simulink model "RADTRANS003"  (R2020b)
settings: Solver=VariableStepAuto  StartTime=0.0  StopTime=10.0  RelTol=1e-3
undefined symbols (not defined in the file): L_street, Line_110_C, Line_110_L, Line_110_R, Line_220_C, Line_220_L, Line_220_R, Line_35_C, Line_35_L, Line_35_R, Line_6_L, Line_6_R, P_nom_dyn, Q_nom_dyn, R_street, Sys_f_Hz, Sys_V_net_kV, Tr_110_35_L_pu, Tr_110_35_R_pu, Tr_110_35_Sn_VA, Tr_110_35_V_HV_kV, Tr_110_35_V_LV_kV, Tr_110_6_L_pu, Tr_110_6_R_pu, Tr_110_6_Sn_VA, Tr_110_6_V_HV_kV, Tr_110_6_V_LV_kV, Tr_220_110_L_pu, Tr_220_110_R_pu, Tr_220_110_Sn_VA, Tr_220_110_V_HV_kV, Tr_220_110_V_LV_kV, Tr_35_04_L_pu, Tr_35_04_R_pu, Tr_35_04_Sn_VA, Tr_35_04_V_HV_kV, Tr_35_04_V_LV_kV, Tr_6_04_L_pu, Tr_6_04_R_pu, Tr_6_04_Sn_VA, Tr_6_04_V_HV_kV, Tr_6_04_V_LV_kV, Ts_powergui
libraries: dspstat3 x96, powerlib x81, powerlib_meascontrol x24, simulink x2
(part 2 of 3)

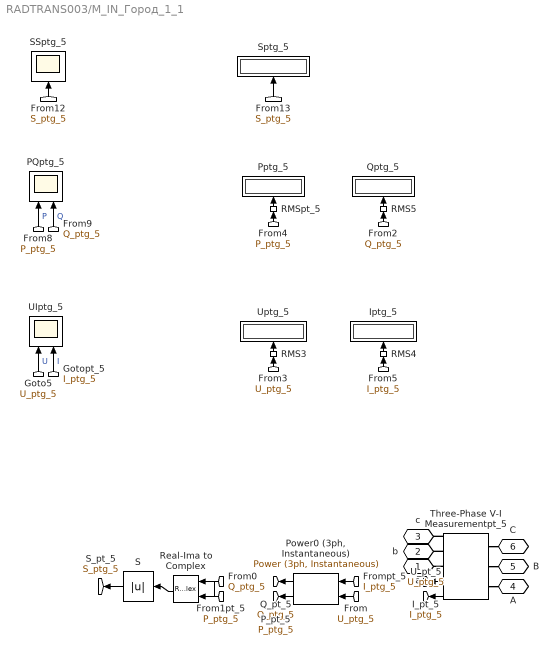
== system RADTRANS003/M_IN_Город_1_1 ==
  Iptg_5 : Display
      settings: Format=bank
  PQptg_5 : Scope  NumInputPorts=2
  "Power0 (3ph, Instantaneous)" : powerlib_meascontrol/Measurements/Power (3ph, Instantaneous)
  Pptg_5 : Display
      settings: Format=bank
  Qptg_5 : Display
      settings: Format=bank
  RMS3 : dspstat3/RMS  run=off  directionMode=Each column  dimension=1  InputProcessing=Columns as channels (frame based)  reset_popup=None
  RMS4 : dspstat3/RMS  run=off  directionMode=Each column  dimension=1  InputProcessing=Columns as channels (frame based)  reset_popup=None
  RMS5 : dspstat3/RMS  run=off  directionMode=Each column  dimension=1  InputProcessing=Columns as channels (frame based)  reset_popup=None
  RMSpt_5 : dspstat3/RMS  run=off  directionMode=Each column  dimension=1  InputProcessing=Columns as channels (frame based)  reset_popup=None
  Real-Ima to Complex : RealImagToComplex
  S : Abs
  SSptg_5 : Scope
  Sptg_5 : Display
      settings: Format=bank
  Three-Phase V-I Measurementpt_5 : powerlib/Measurements/Three-Phase V-I Measurement  VoltageMeasurement=phase-to-ground  SetLabelV=off  LabelV=Vabc  Vpu=off  VpuLL=off  CurrentMeasurement=yes  SetLabelI=off  LabelI=Iabc  Ipu=off  Pbase=100e6  Vbase=500e3  OutputType=Complex  PhasorSimulation=off  PSBequivalent=0
  UIptg_5 : Scope  NumInputPorts=2
  Uptg_5 : Display
      settings: Format=bank
  a : PMIOPort  Side=Right
  b : PMIOPort  Port=2  Side=Right
  c : PMIOPort  Port=3  Side=Right
  A : PMIOPort  Port=4  Side=Left
  B : PMIOPort  Port=5  Side=Left
  C : PMIOPort  Port=6  Side=Left
  tag scope: I_ptg_5=global, P_ptg_5=global, Q_ptg_5=global, S_ptg_5=global, U_ptg_5=global
  wires:
  S/1 -> [S_ptg_5]
  Real-Ima to Complex/1 -> S/1
  [S_ptg_5] -> Sptg_5/1
  [S_ptg_5] -> SSptg_5/1
  [P_ptg_5] -> RMSpt_5/1
  RMSpt_5/1 -> Pptg_5/1
  RMS5/1 -> Qptg_5/1
  [U_ptg_5] -> RMS3/1
  RMS3/1 -> Uptg_5/1
  [P_ptg_5] -> Real-Ima to Complex/1
  [Q_ptg_5] -> RMS5/1
  [I_ptg_5] -> RMS4/1
  RMS4/1 -> Iptg_5/1
  [U_ptg_5] -> UIptg_5/1  "U"
  [P_ptg_5] -> PQptg_5/1  "P"
  [I_ptg_5] -> UIptg_5/2  "I"
  Three-Phase V-I Measurementpt_5/1 -> [U_ptg_5]
  [Q_ptg_5] -> Real-Ima to Complex/2
  Three-Phase V-I Measurementpt_5/2 -> [I_ptg_5]
  [U_ptg_5] -> "Power0 (3ph, Instantaneous)"/1
  [I_ptg_5] -> "Power0 (3ph, Instantaneous)"/2
  "Power0 (3ph, Instantaneous)"/2 -> [Q_ptg_5]
  "Power0 (3ph, Instantaneous)"/1 -> [P_ptg_5]
  [Q_ptg_5] -> PQptg_5/2  "Q"
  connections:
  Three-Phase V-I Measurementpt_5/LConn1 -- A/RConn1
  Three-Phase V-I Measurementpt_5/RConn1 -- a/RConn1
  Three-Phase V-I Measurementpt_5/LConn2 -- B/RConn1
  Three-Phase V-I Measurementpt_5/LConn3 -- C/RConn1
  Three-Phase V-I Measurementpt_5/RConn3 -- c/RConn1
  Three-Phase V-I Measurementpt_5/RConn2 -- b/RConn1

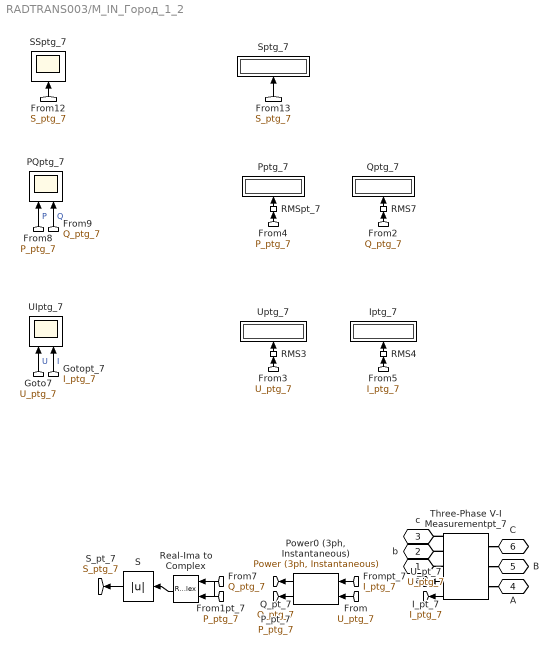
== system RADTRANS003/M_IN_Город_1_2 ==
  Iptg_7 : Display
      settings: Format=bank
  PQptg_7 : Scope  NumInputPorts=2
  "Power0 (3ph, Instantaneous)" : powerlib_meascontrol/Measurements/Power (3ph, Instantaneous)
  Pptg_7 : Display
      settings: Format=bank
  Qptg_7 : Display
      settings: Format=bank
  RMS3 : dspstat3/RMS  run=off  directionMode=Each column  dimension=1  InputProcessing=Columns as channels (frame based)  reset_popup=None
  RMS4 : dspstat3/RMS  run=off  directionMode=Each column  dimension=1  InputProcessing=Columns as channels (frame based)  reset_popup=None
  RMS7 : dspstat3/RMS  run=off  directionMode=Each column  dimension=1  InputProcessing=Columns as channels (frame based)  reset_popup=None
  RMSpt_7 : dspstat3/RMS  run=off  directionMode=Each column  dimension=1  InputProcessing=Columns as channels (frame based)  reset_popup=None
  Real-Ima to Complex : RealImagToComplex
  S : Abs
  SSptg_7 : Scope
  Sptg_7 : Display
      settings: Format=bank
  Three-Phase V-I Measurementpt_7 : powerlib/Measurements/Three-Phase V-I Measurement  VoltageMeasurement=phase-to-ground  SetLabelV=off  LabelV=Vabc  Vpu=off  VpuLL=off  CurrentMeasurement=yes  SetLabelI=off  LabelI=Iabc  Ipu=off  Pbase=100e6  Vbase=500e3  OutputType=Complex  PhasorSimulation=off  PSBequivalent=0
  UIptg_7 : Scope  NumInputPorts=2
  Uptg_7 : Display
      settings: Format=bank
  a : PMIOPort  Side=Right
  b : PMIOPort  Port=2  Side=Right
  c : PMIOPort  Port=3  Side=Right
  A : PMIOPort  Port=4  Side=Left
  B : PMIOPort  Port=5  Side=Left
  C : PMIOPort  Port=6  Side=Left
  tag scope: I_ptg_7=global, P_ptg_7=global, Q_ptg_7=global, S_ptg_7=global, U_ptg_7=global
  wires:
  S/1 -> [S_ptg_7]
  Real-Ima to Complex/1 -> S/1
  [S_ptg_7] -> Sptg_7/1
  [S_ptg_7] -> SSptg_7/1
  [P_ptg_7] -> RMSpt_7/1
  RMSpt_7/1 -> Pptg_7/1
  RMS7/1 -> Qptg_7/1
  [U_ptg_7] -> RMS3/1
  RMS3/1 -> Uptg_7/1
  [P_ptg_7] -> Real-Ima to Complex/1
  [Q_ptg_7] -> RMS7/1
  [I_ptg_7] -> RMS4/1
  RMS4/1 -> Iptg_7/1
  [U_ptg_7] -> UIptg_7/1  "U"
  [P_ptg_7] -> PQptg_7/1  "P"
  [I_ptg_7] -> UIptg_7/2  "I"
  Three-Phase V-I Measurementpt_7/1 -> [U_ptg_7]
  [Q_ptg_7] -> Real-Ima to Complex/2
  Three-Phase V-I Measurementpt_7/2 -> [I_ptg_7]
  [U_ptg_7] -> "Power0 (3ph, Instantaneous)"/1
  [I_ptg_7] -> "Power0 (3ph, Instantaneous)"/2
  "Power0 (3ph, Instantaneous)"/2 -> [Q_ptg_7]
  "Power0 (3ph, Instantaneous)"/1 -> [P_ptg_7]
  [Q_ptg_7] -> PQptg_7/2  "Q"
  connections:
  Three-Phase V-I Measurementpt_7/LConn1 -- A/RConn1
  Three-Phase V-I Measurementpt_7/RConn1 -- a/RConn1
  Three-Phase V-I Measurementpt_7/LConn2 -- B/RConn1
  Three-Phase V-I Measurementpt_7/LConn3 -- C/RConn1
  Three-Phase V-I Measurementpt_7/RConn3 -- c/RConn1
  Three-Phase V-I Measurementpt_7/RConn2 -- b/RConn1

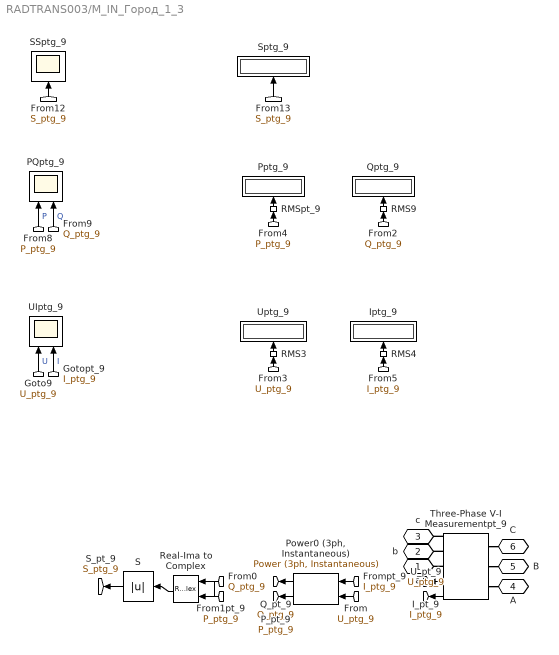
== system RADTRANS003/M_IN_Город_1_3 ==
  Iptg_9 : Display
      settings: Format=bank
  PQptg_9 : Scope  NumInputPorts=2
  "Power0 (3ph, Instantaneous)" : powerlib_meascontrol/Measurements/Power (3ph, Instantaneous)
  Pptg_9 : Display
      settings: Format=bank
  Qptg_9 : Display
      settings: Format=bank
  RMS3 : dspstat3/RMS  run=off  directionMode=Each column  dimension=1  InputProcessing=Columns as channels (frame based)  reset_popup=None
  RMS4 : dspstat3/RMS  run=off  directionMode=Each column  dimension=1  InputProcessing=Columns as channels (frame based)  reset_popup=None
  RMS9 : dspstat3/RMS  run=off  directionMode=Each column  dimension=1  InputProcessing=Columns as channels (frame based)  reset_popup=None
  RMSpt_9 : dspstat3/RMS  run=off  directionMode=Each column  dimension=1  InputProcessing=Columns as channels (frame based)  reset_popup=None
  Real-Ima to Complex : RealImagToComplex
  S : Abs
  SSptg_9 : Scope
  Sptg_9 : Display
      settings: Format=bank
  Three-Phase V-I Measurementpt_9 : powerlib/Measurements/Three-Phase V-I Measurement  VoltageMeasurement=phase-to-ground  SetLabelV=off  LabelV=Vabc  Vpu=off  VpuLL=off  CurrentMeasurement=yes  SetLabelI=off  LabelI=Iabc  Ipu=off  Pbase=100e6  Vbase=500e3  OutputType=Complex  PhasorSimulation=off  PSBequivalent=0
  UIptg_9 : Scope  NumInputPorts=2
  Uptg_9 : Display
      settings: Format=bank
  a : PMIOPort  Side=Right
  b : PMIOPort  Port=2  Side=Right
  c : PMIOPort  Port=3  Side=Right
  A : PMIOPort  Port=4  Side=Left
  B : PMIOPort  Port=5  Side=Left
  C : PMIOPort  Port=6  Side=Left
  tag scope: I_ptg_9=global, P_ptg_9=global, Q_ptg_9=global, S_ptg_9=global, U_ptg_9=global
  wires:
  S/1 -> [S_ptg_9]
  Real-Ima to Complex/1 -> S/1
  [S_ptg_9] -> Sptg_9/1
  [S_ptg_9] -> SSptg_9/1
  [P_ptg_9] -> RMSpt_9/1
  RMSpt_9/1 -> Pptg_9/1
  RMS9/1 -> Qptg_9/1
  [U_ptg_9] -> RMS3/1
  RMS3/1 -> Uptg_9/1
  [P_ptg_9] -> Real-Ima to Complex/1
  [Q_ptg_9] -> RMS9/1
  [I_ptg_9] -> RMS4/1
  RMS4/1 -> Iptg_9/1
  [U_ptg_9] -> UIptg_9/1  "U"
  [P_ptg_9] -> PQptg_9/1  "P"
  [I_ptg_9] -> UIptg_9/2  "I"
  Three-Phase V-I Measurementpt_9/1 -> [U_ptg_9]
  [Q_ptg_9] -> Real-Ima to Complex/2
  Three-Phase V-I Measurementpt_9/2 -> [I_ptg_9]
  [U_ptg_9] -> "Power0 (3ph, Instantaneous)"/1
  [I_ptg_9] -> "Power0 (3ph, Instantaneous)"/2
  "Power0 (3ph, Instantaneous)"/2 -> [Q_ptg_9]
  "Power0 (3ph, Instantaneous)"/1 -> [P_ptg_9]
  [Q_ptg_9] -> PQptg_9/2  "Q"
  connections:
  Three-Phase V-I Measurementpt_9/LConn1 -- A/RConn1
  Three-Phase V-I Measurementpt_9/RConn1 -- a/RConn1
  Three-Phase V-I Measurementpt_9/LConn2 -- B/RConn1
  Three-Phase V-I Measurementpt_9/LConn3 -- C/RConn1
  Three-Phase V-I Measurementpt_9/RConn3 -- c/RConn1
  Three-Phase V-I Measurementpt_9/RConn2 -- b/RConn1

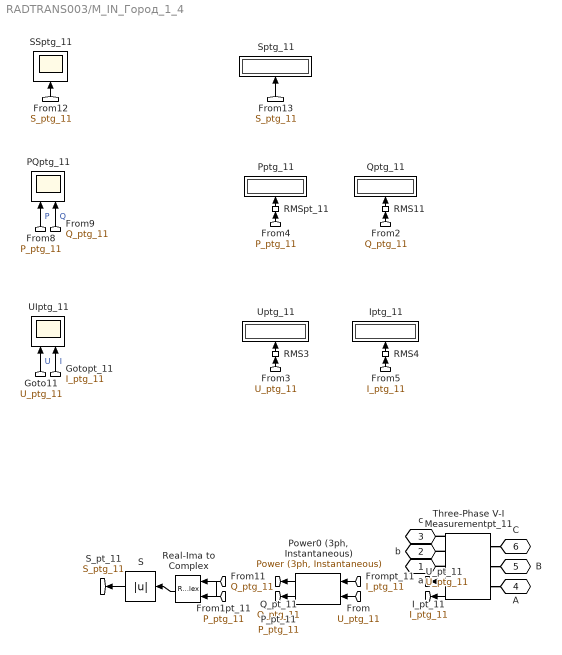
== system RADTRANS003/M_IN_Город_1_4 ==
  Iptg_11 : Display
      settings: Format=bank
  PQptg_11 : Scope  NumInputPorts=2
  "Power0 (3ph, Instantaneous)" : powerlib_meascontrol/Measurements/Power (3ph, Instantaneous)
  Pptg_11 : Display
      settings: Format=bank
  Qptg_11 : Display
      settings: Format=bank
  RMS11 : dspstat3/RMS  run=off  directionMode=Each column  dimension=1  InputProcessing=Columns as channels (frame based)  reset_popup=None
  RMS3 : dspstat3/RMS  run=off  directionMode=Each column  dimension=1  InputProcessing=Columns as channels (frame based)  reset_popup=None
  RMS4 : dspstat3/RMS  run=off  directionMode=Each column  dimension=1  InputProcessing=Columns as channels (frame based)  reset_popup=None
  RMSpt_11 : dspstat3/RMS  run=off  directionMode=Each column  dimension=1  InputProcessing=Columns as channels (frame based)  reset_popup=None
  Real-Ima to Complex : RealImagToComplex
  S : Abs
  SSptg_11 : Scope
  Sptg_11 : Display
      settings: Format=bank
  Three-Phase V-I Measurementpt_11 : powerlib/Measurements/Three-Phase V-I Measurement  VoltageMeasurement=phase-to-ground  SetLabelV=off  LabelV=Vabc  Vpu=off  VpuLL=off  CurrentMeasurement=yes  SetLabelI=off  LabelI=Iabc  Ipu=off  Pbase=100e6  Vbase=500e3  OutputType=Complex  PhasorSimulation=off  PSBequivalent=0
  UIptg_11 : Scope  NumInputPorts=2
  Uptg_11 : Display
      settings: Format=bank
  a : PMIOPort  Side=Right
  b : PMIOPort  Port=2  Side=Right
  c : PMIOPort  Port=3  Side=Right
  A : PMIOPort  Port=4  Side=Left
  B : PMIOPort  Port=5  Side=Left
  C : PMIOPort  Port=6  Side=Left
  tag scope: I_ptg_11=global, P_ptg_11=global, Q_ptg_11=global, S_ptg_11=global, U_ptg_11=global
  wires:
  S/1 -> [S_ptg_11]
  Real-Ima to Complex/1 -> S/1
  [S_ptg_11] -> Sptg_11/1
  [S_ptg_11] -> SSptg_11/1
  [P_ptg_11] -> RMSpt_11/1
  RMSpt_11/1 -> Pptg_11/1
  RMS11/1 -> Qptg_11/1
  [U_ptg_11] -> RMS3/1
  RMS3/1 -> Uptg_11/1
  [P_ptg_11] -> Real-Ima to Complex/1
  [Q_ptg_11] -> RMS11/1
  [I_ptg_11] -> RMS4/1
  RMS4/1 -> Iptg_11/1
  [U_ptg_11] -> UIptg_11/1  "U"
  [P_ptg_11] -> PQptg_11/1  "P"
  [I_ptg_11] -> UIptg_11/2  "I"
  Three-Phase V-I Measurementpt_11/1 -> [U_ptg_11]
  [Q_ptg_11] -> Real-Ima to Complex/2
  Three-Phase V-I Measurementpt_11/2 -> [I_ptg_11]
  [U_ptg_11] -> "Power0 (3ph, Instantaneous)"/1
  [I_ptg_11] -> "Power0 (3ph, Instantaneous)"/2
  "Power0 (3ph, Instantaneous)"/2 -> [Q_ptg_11]
  "Power0 (3ph, Instantaneous)"/1 -> [P_ptg_11]
  [Q_ptg_11] -> PQptg_11/2  "Q"
  connections:
  Three-Phase V-I Measurementpt_11/LConn1 -- A/RConn1
  Three-Phase V-I Measurementpt_11/RConn1 -- a/RConn1
  Three-Phase V-I Measurementpt_11/LConn2 -- B/RConn1
  Three-Phase V-I Measurementpt_11/LConn3 -- C/RConn1
  Three-Phase V-I Measurementpt_11/RConn3 -- c/RConn1
  Three-Phase V-I Measurementpt_11/RConn2 -- b/RConn1

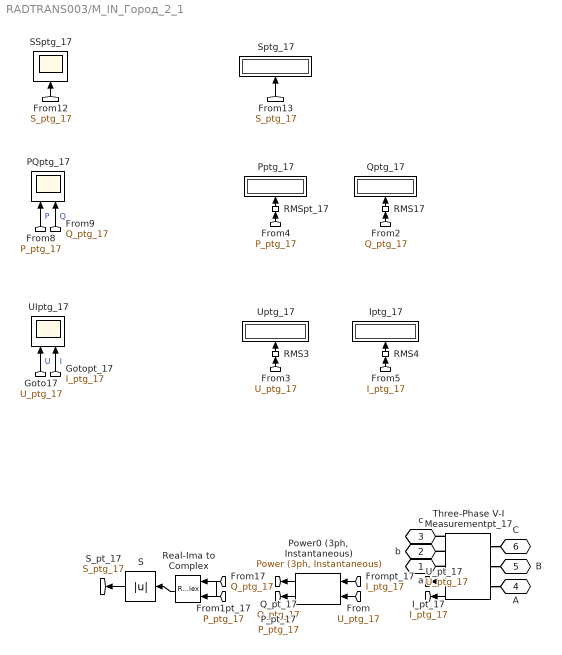
== system RADTRANS003/M_IN_Город_2_1 ==
  Iptg_17 : Display
      settings: Format=bank
  PQptg_17 : Scope  NumInputPorts=2
  "Power0 (3ph, Instantaneous)" : powerlib_meascontrol/Measurements/Power (3ph, Instantaneous)
  Pptg_17 : Display
      settings: Format=bank
  Qptg_17 : Display
      settings: Format=bank
  RMS17 : dspstat3/RMS  run=off  directionMode=Each column  dimension=1  InputProcessing=Columns as channels (frame based)  reset_popup=None
  RMS3 : dspstat3/RMS  run=off  directionMode=Each column  dimension=1  InputProcessing=Columns as channels (frame based)  reset_popup=None
  RMS4 : dspstat3/RMS  run=off  directionMode=Each column  dimension=1  InputProcessing=Columns as channels (frame based)  reset_popup=None
  RMSpt_17 : dspstat3/RMS  run=off  directionMode=Each column  dimension=1  InputProcessing=Columns as channels (frame based)  reset_popup=None
  Real-Ima to Complex : RealImagToComplex
  S : Abs
  SSptg_17 : Scope
  Sptg_17 : Display
      settings: Format=bank
  Three-Phase V-I Measurementpt_17 : powerlib/Measurements/Three-Phase V-I Measurement  VoltageMeasurement=phase-to-ground  SetLabelV=off  LabelV=Vabc  Vpu=off  VpuLL=off  CurrentMeasurement=yes  SetLabelI=off  LabelI=Iabc  Ipu=off  Pbase=100e6  Vbase=500e3  OutputType=Complex  PhasorSimulation=off  PSBequivalent=0
  UIptg_17 : Scope  NumInputPorts=2
  Uptg_17 : Display
      settings: Format=bank
  a : PMIOPort  Side=Right
  b : PMIOPort  Port=2  Side=Right
  c : PMIOPort  Port=3  Side=Right
  A : PMIOPort  Port=4  Side=Left
  B : PMIOPort  Port=5  Side=Left
  C : PMIOPort  Port=6  Side=Left
  tag scope: I_ptg_17=global, P_ptg_17=global, Q_ptg_17=global, S_ptg_17=global, U_ptg_17=global
  wires:
  S/1 -> [S_ptg_17]
  Real-Ima to Complex/1 -> S/1
  [S_ptg_17] -> Sptg_17/1
  [S_ptg_17] -> SSptg_17/1
  [P_ptg_17] -> RMSpt_17/1
  RMSpt_17/1 -> Pptg_17/1
  RMS17/1 -> Qptg_17/1
  [U_ptg_17] -> RMS3/1
  RMS3/1 -> Uptg_17/1
  [P_ptg_17] -> Real-Ima to Complex/1
  [Q_ptg_17] -> RMS17/1
  [I_ptg_17] -> RMS4/1
  RMS4/1 -> Iptg_17/1
  [U_ptg_17] -> UIptg_17/1  "U"
  [P_ptg_17] -> PQptg_17/1  "P"
  [I_ptg_17] -> UIptg_17/2  "I"
  Three-Phase V-I Measurementpt_17/1 -> [U_ptg_17]
  [Q_ptg_17] -> Real-Ima to Complex/2
  Three-Phase V-I Measurementpt_17/2 -> [I_ptg_17]
  [U_ptg_17] -> "Power0 (3ph, Instantaneous)"/1
  [I_ptg_17] -> "Power0 (3ph, Instantaneous)"/2
  "Power0 (3ph, Instantaneous)"/2 -> [Q_ptg_17]
  "Power0 (3ph, Instantaneous)"/1 -> [P_ptg_17]
  [Q_ptg_17] -> PQptg_17/2  "Q"
  connections:
  Three-Phase V-I Measurementpt_17/LConn1 -- A/RConn1
  Three-Phase V-I Measurementpt_17/RConn1 -- a/RConn1
  Three-Phase V-I Measurementpt_17/LConn2 -- B/RConn1
  Three-Phase V-I Measurementpt_17/LConn3 -- C/RConn1
  Three-Phase V-I Measurementpt_17/RConn3 -- c/RConn1
  Three-Phase V-I Measurementpt_17/RConn2 -- b/RConn1

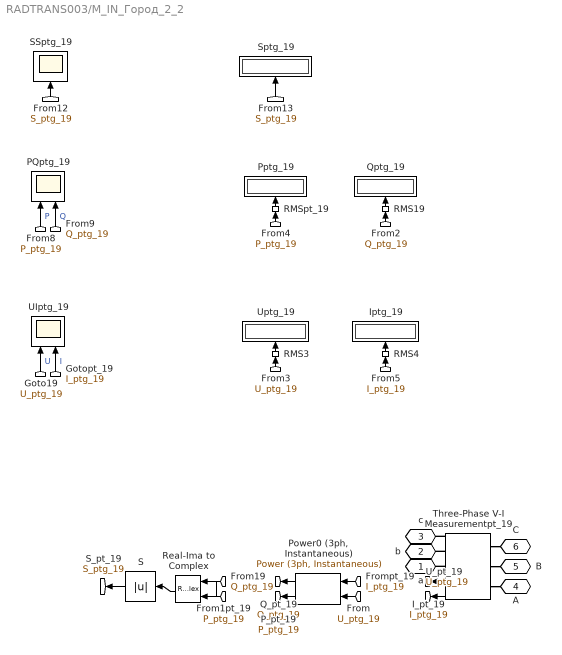
== system RADTRANS003/M_IN_Город_2_2 ==
  Iptg_19 : Display
      settings: Format=bank
  PQptg_19 : Scope  NumInputPorts=2
  "Power0 (3ph, Instantaneous)" : powerlib_meascontrol/Measurements/Power (3ph, Instantaneous)
  Pptg_19 : Display
      settings: Format=bank
  Qptg_19 : Display
      settings: Format=bank
  RMS19 : dspstat3/RMS  run=off  directionMode=Each column  dimension=1  InputProcessing=Columns as channels (frame based)  reset_popup=None
  RMS3 : dspstat3/RMS  run=off  directionMode=Each column  dimension=1  InputProcessing=Columns as channels (frame based)  reset_popup=None
  RMS4 : dspstat3/RMS  run=off  directionMode=Each column  dimension=1  InputProcessing=Columns as channels (frame based)  reset_popup=None
  RMSpt_19 : dspstat3/RMS  run=off  directionMode=Each column  dimension=1  InputProcessing=Columns as channels (frame based)  reset_popup=None
  Real-Ima to Complex : RealImagToComplex
  S : Abs
  SSptg_19 : Scope
  Sptg_19 : Display
      settings: Format=bank
  Three-Phase V-I Measurementpt_19 : powerlib/Measurements/Three-Phase V-I Measurement  VoltageMeasurement=phase-to-ground  SetLabelV=off  LabelV=Vabc  Vpu=off  VpuLL=off  CurrentMeasurement=yes  SetLabelI=off  LabelI=Iabc  Ipu=off  Pbase=100e6  Vbase=500e3  OutputType=Complex  PhasorSimulation=off  PSBequivalent=0
  UIptg_19 : Scope  NumInputPorts=2
  Uptg_19 : Display
      settings: Format=bank
  a : PMIOPort  Side=Right
  b : PMIOPort  Port=2  Side=Right
  c : PMIOPort  Port=3  Side=Right
  A : PMIOPort  Port=4  Side=Left
  B : PMIOPort  Port=5  Side=Left
  C : PMIOPort  Port=6  Side=Left
  tag scope: I_ptg_19=global, P_ptg_19=global, Q_ptg_19=global, S_ptg_19=global, U_ptg_19=global
  wires:
  S/1 -> [S_ptg_19]
  Real-Ima to Complex/1 -> S/1
  [S_ptg_19] -> Sptg_19/1
  [S_ptg_19] -> SSptg_19/1
  [P_ptg_19] -> RMSpt_19/1
  RMSpt_19/1 -> Pptg_19/1
  RMS19/1 -> Qptg_19/1
  [U_ptg_19] -> RMS3/1
  RMS3/1 -> Uptg_19/1
  [P_ptg_19] -> Real-Ima to Complex/1
  [Q_ptg_19] -> RMS19/1
  [I_ptg_19] -> RMS4/1
  RMS4/1 -> Iptg_19/1
  [U_ptg_19] -> UIptg_19/1  "U"
  [P_ptg_19] -> PQptg_19/1  "P"
  [I_ptg_19] -> UIptg_19/2  "I"
  Three-Phase V-I Measurementpt_19/1 -> [U_ptg_19]
  [Q_ptg_19] -> Real-Ima to Complex/2
  Three-Phase V-I Measurementpt_19/2 -> [I_ptg_19]
  [U_ptg_19] -> "Power0 (3ph, Instantaneous)"/1
  [I_ptg_19] -> "Power0 (3ph, Instantaneous)"/2
  "Power0 (3ph, Instantaneous)"/2 -> [Q_ptg_19]
  "Power0 (3ph, Instantaneous)"/1 -> [P_ptg_19]
  [Q_ptg_19] -> PQptg_19/2  "Q"
  connections:
  Three-Phase V-I Measurementpt_19/LConn1 -- A/RConn1
  Three-Phase V-I Measurementpt_19/RConn1 -- a/RConn1
  Three-Phase V-I Measurementpt_19/LConn2 -- B/RConn1
  Three-Phase V-I Measurementpt_19/LConn3 -- C/RConn1
  Three-Phase V-I Measurementpt_19/RConn3 -- c/RConn1
  Three-Phase V-I Measurementpt_19/RConn2 -- b/RConn1

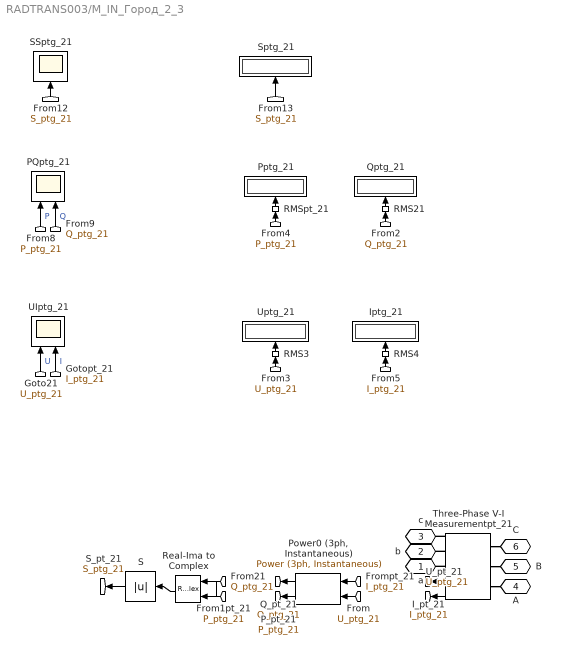
== system RADTRANS003/M_IN_Город_2_3 ==
  Iptg_21 : Display
      settings: Format=bank
  PQptg_21 : Scope  NumInputPorts=2
  "Power0 (3ph, Instantaneous)" : powerlib_meascontrol/Measurements/Power (3ph, Instantaneous)
  Pptg_21 : Display
      settings: Format=bank
  Qptg_21 : Display
      settings: Format=bank
  RMS21 : dspstat3/RMS  run=off  directionMode=Each column  dimension=1  InputProcessing=Columns as channels (frame based)  reset_popup=None
  RMS3 : dspstat3/RMS  run=off  directionMode=Each column  dimension=1  InputProcessing=Columns as channels (frame based)  reset_popup=None
  RMS4 : dspstat3/RMS  run=off  directionMode=Each column  dimension=1  InputProcessing=Columns as channels (frame based)  reset_popup=None
  RMSpt_21 : dspstat3/RMS  run=off  directionMode=Each column  dimension=1  InputProcessing=Columns as channels (frame based)  reset_popup=None
  Real-Ima to Complex : RealImagToComplex
  S : Abs
  SSptg_21 : Scope
  Sptg_21 : Display
      settings: Format=bank
  Three-Phase V-I Measurementpt_21 : powerlib/Measurements/Three-Phase V-I Measurement  VoltageMeasurement=phase-to-ground  SetLabelV=off  LabelV=Vabc  Vpu=off  VpuLL=off  CurrentMeasurement=yes  SetLabelI=off  LabelI=Iabc  Ipu=off  Pbase=100e6  Vbase=500e3  OutputType=Complex  PhasorSimulation=off  PSBequivalent=0
  UIptg_21 : Scope  NumInputPorts=2
  Uptg_21 : Display
      settings: Format=bank
  a : PMIOPort  Side=Right
  b : PMIOPort  Port=2  Side=Right
  c : PMIOPort  Port=3  Side=Right
  A : PMIOPort  Port=4  Side=Left
  B : PMIOPort  Port=5  Side=Left
  C : PMIOPort  Port=6  Side=Left
  tag scope: I_ptg_21=global, P_ptg_21=global, Q_ptg_21=global, S_ptg_21=global, U_ptg_21=global
  wires:
  S/1 -> [S_ptg_21]
  Real-Ima to Complex/1 -> S/1
  [S_ptg_21] -> Sptg_21/1
  [S_ptg_21] -> SSptg_21/1
  [P_ptg_21] -> RMSpt_21/1
  RMSpt_21/1 -> Pptg_21/1
  RMS21/1 -> Qptg_21/1
  [U_ptg_21] -> RMS3/1
  RMS3/1 -> Uptg_21/1
  [P_ptg_21] -> Real-Ima to Complex/1
  [Q_ptg_21] -> RMS21/1
  [I_ptg_21] -> RMS4/1
  RMS4/1 -> Iptg_21/1
  [U_ptg_21] -> UIptg_21/1  "U"
  [P_ptg_21] -> PQptg_21/1  "P"
  [I_ptg_21] -> UIptg_21/2  "I"
  Three-Phase V-I Measurementpt_21/1 -> [U_ptg_21]
  [Q_ptg_21] -> Real-Ima to Complex/2
  Three-Phase V-I Measurementpt_21/2 -> [I_ptg_21]
  [U_ptg_21] -> "Power0 (3ph, Instantaneous)"/1
  [I_ptg_21] -> "Power0 (3ph, Instantaneous)"/2
  "Power0 (3ph, Instantaneous)"/2 -> [Q_ptg_21]
  "Power0 (3ph, Instantaneous)"/1 -> [P_ptg_21]
  [Q_ptg_21] -> PQptg_21/2  "Q"
  connections:
  Three-Phase V-I Measurementpt_21/LConn1 -- A/RConn1
  Three-Phase V-I Measurementpt_21/RConn1 -- a/RConn1
  Three-Phase V-I Measurementpt_21/LConn2 -- B/RConn1
  Three-Phase V-I Measurementpt_21/LConn3 -- C/RConn1
  Three-Phase V-I Measurementpt_21/RConn3 -- c/RConn1
  Three-Phase V-I Measurementpt_21/RConn2 -- b/RConn1

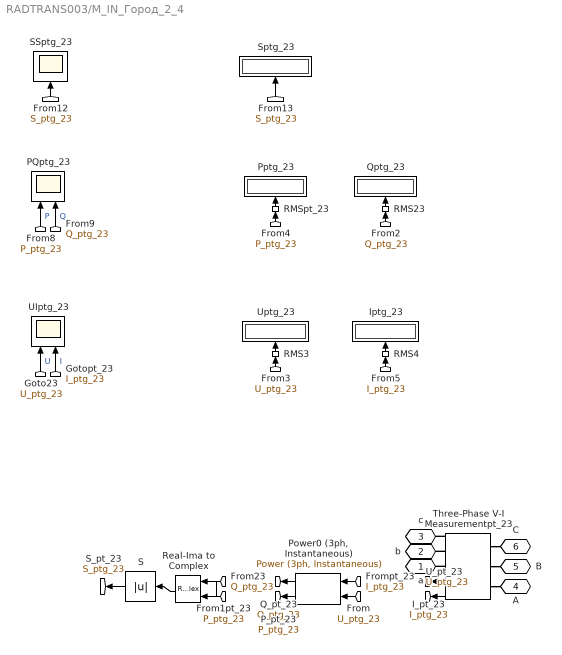
== system RADTRANS003/M_IN_Город_2_4 ==
  Iptg_23 : Display
      settings: Format=bank
  PQptg_23 : Scope  NumInputPorts=2
  "Power0 (3ph, Instantaneous)" : powerlib_meascontrol/Measurements/Power (3ph, Instantaneous)
  Pptg_23 : Display
      settings: Format=bank
  Qptg_23 : Display
      settings: Format=bank
  RMS23 : dspstat3/RMS  run=off  directionMode=Each column  dimension=1  InputProcessing=Columns as channels (frame based)  reset_popup=None
  RMS3 : dspstat3/RMS  run=off  directionMode=Each column  dimension=1  InputProcessing=Columns as channels (frame based)  reset_popup=None
  RMS4 : dspstat3/RMS  run=off  directionMode=Each column  dimension=1  InputProcessing=Columns as channels (frame based)  reset_popup=None
  RMSpt_23 : dspstat3/RMS  run=off  directionMode=Each column  dimension=1  InputProcessing=Columns as channels (frame based)  reset_popup=None
  Real-Ima to Complex : RealImagToComplex
  S : Abs
  SSptg_23 : Scope
  Sptg_23 : Display
      settings: Format=bank
  Three-Phase V-I Measurementpt_23 : powerlib/Measurements/Three-Phase V-I Measurement  VoltageMeasurement=phase-to-ground  SetLabelV=off  LabelV=Vabc  Vpu=off  VpuLL=off  CurrentMeasurement=yes  SetLabelI=off  LabelI=Iabc  Ipu=off  Pbase=100e6  Vbase=500e3  OutputType=Complex  PhasorSimulation=off  PSBequivalent=0
  UIptg_23 : Scope  NumInputPorts=2
  Uptg_23 : Display
      settings: Format=bank
  a : PMIOPort  Side=Right
  b : PMIOPort  Port=2  Side=Right
  c : PMIOPort  Port=3  Side=Right
  A : PMIOPort  Port=4  Side=Left
  B : PMIOPort  Port=5  Side=Left
  C : PMIOPort  Port=6  Side=Left
  tag scope: I_ptg_23=global, P_ptg_23=global, Q_ptg_23=global, S_ptg_23=global, U_ptg_23=global
  wires:
  S/1 -> [S_ptg_23]
  Real-Ima to Complex/1 -> S/1
  [S_ptg_23] -> Sptg_23/1
  [S_ptg_23] -> SSptg_23/1
  [P_ptg_23] -> RMSpt_23/1
  RMSpt_23/1 -> Pptg_23/1
  RMS23/1 -> Qptg_23/1
  [U_ptg_23] -> RMS3/1
  RMS3/1 -> Uptg_23/1
  [P_ptg_23] -> Real-Ima to Complex/1
  [Q_ptg_23] -> RMS23/1
  [I_ptg_23] -> RMS4/1
  RMS4/1 -> Iptg_23/1
  [U_ptg_23] -> UIptg_23/1  "U"
  [P_ptg_23] -> PQptg_23/1  "P"
  [I_ptg_23] -> UIptg_23/2  "I"
  Three-Phase V-I Measurementpt_23/1 -> [U_ptg_23]
  [Q_ptg_23] -> Real-Ima to Complex/2
  Three-Phase V-I Measurementpt_23/2 -> [I_ptg_23]
  [U_ptg_23] -> "Power0 (3ph, Instantaneous)"/1
  [I_ptg_23] -> "Power0 (3ph, Instantaneous)"/2
  "Power0 (3ph, Instantaneous)"/2 -> [Q_ptg_23]
  "Power0 (3ph, Instantaneous)"/1 -> [P_ptg_23]
  [Q_ptg_23] -> PQptg_23/2  "Q"
  connections:
  Three-Phase V-I Measurementpt_23/LConn1 -- A/RConn1
  Three-Phase V-I Measurementpt_23/RConn1 -- a/RConn1
  Three-Phase V-I Measurementpt_23/LConn2 -- B/RConn1
  Three-Phase V-I Measurementpt_23/LConn3 -- C/RConn1
  Three-Phase V-I Measurementpt_23/RConn3 -- c/RConn1
  Three-Phase V-I Measurementpt_23/RConn2 -- b/RConn1

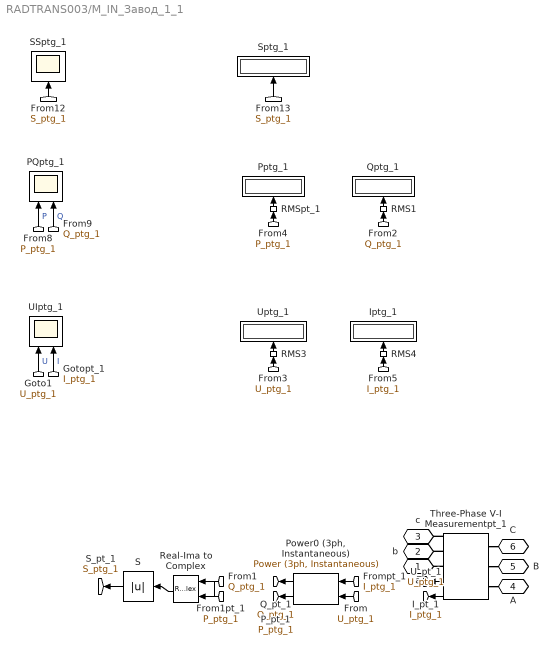
== system RADTRANS003/M_IN_Завод_1_1 ==
  Iptg_1 : Display
      settings: Format=bank
  PQptg_1 : Scope  NumInputPorts=2
  "Power0 (3ph, Instantaneous)" : powerlib_meascontrol/Measurements/Power (3ph, Instantaneous)
  Pptg_1 : Display
      settings: Format=bank
  Qptg_1 : Display
      settings: Format=bank
  RMS1 : dspstat3/RMS  run=off  directionMode=Each column  dimension=1  InputProcessing=Columns as channels (frame based)  reset_popup=None
  RMS3 : dspstat3/RMS  run=off  directionMode=Each column  dimension=1  InputProcessing=Columns as channels (frame based)  reset_popup=None
  RMS4 : dspstat3/RMS  run=off  directionMode=Each column  dimension=1  InputProcessing=Columns as channels (frame based)  reset_popup=None
  RMSpt_1 : dspstat3/RMS  run=off  directionMode=Each column  dimension=1  InputProcessing=Columns as channels (frame based)  reset_popup=None
  Real-Ima to Complex : RealImagToComplex
  S : Abs
  SSptg_1 : Scope
  Sptg_1 : Display
      settings: Format=bank
  Three-Phase V-I Measurementpt_1 : powerlib/Measurements/Three-Phase V-I Measurement  VoltageMeasurement=phase-to-ground  SetLabelV=off  LabelV=Vabc  Vpu=off  VpuLL=off  CurrentMeasurement=yes  SetLabelI=off  LabelI=Iabc  Ipu=off  Pbase=100e6  Vbase=500e3  OutputType=Complex  PhasorSimulation=off  PSBequivalent=0
  UIptg_1 : Scope  NumInputPorts=2
  Uptg_1 : Display
      settings: Format=bank
  a : PMIOPort  Side=Right
  b : PMIOPort  Port=2  Side=Right
  c : PMIOPort  Port=3  Side=Right
  A : PMIOPort  Port=4  Side=Left
  B : PMIOPort  Port=5  Side=Left
  C : PMIOPort  Port=6  Side=Left
  tag scope: I_ptg_1=global, P_ptg_1=global, Q_ptg_1=global, S_ptg_1=global, U_ptg_1=global
  wires:
  S/1 -> [S_ptg_1]
  Real-Ima to Complex/1 -> S/1
  [S_ptg_1] -> Sptg_1/1
  [S_ptg_1] -> SSptg_1/1
  [P_ptg_1] -> RMSpt_1/1
  RMSpt_1/1 -> Pptg_1/1
  RMS1/1 -> Qptg_1/1
  [U_ptg_1] -> RMS3/1
  RMS3/1 -> Uptg_1/1
  [P_ptg_1] -> Real-Ima to Complex/1
  [Q_ptg_1] -> RMS1/1
  [I_ptg_1] -> RMS4/1
  RMS4/1 -> Iptg_1/1
  [U_ptg_1] -> UIptg_1/1  "U"
  [P_ptg_1] -> PQptg_1/1  "P"
  [I_ptg_1] -> UIptg_1/2  "I"
  Three-Phase V-I Measurementpt_1/1 -> [U_ptg_1]
  [Q_ptg_1] -> Real-Ima to Complex/2
  Three-Phase V-I Measurementpt_1/2 -> [I_ptg_1]
  [U_ptg_1] -> "Power0 (3ph, Instantaneous)"/1
  [I_ptg_1] -> "Power0 (3ph, Instantaneous)"/2
  "Power0 (3ph, Instantaneous)"/2 -> [Q_ptg_1]
  "Power0 (3ph, Instantaneous)"/1 -> [P_ptg_1]
  [Q_ptg_1] -> PQptg_1/2  "Q"
  connections:
  Three-Phase V-I Measurementpt_1/LConn1 -- A/RConn1
  Three-Phase V-I Measurementpt_1/RConn1 -- a/RConn1
  Three-Phase V-I Measurementpt_1/LConn2 -- B/RConn1
  Three-Phase V-I Measurementpt_1/LConn3 -- C/RConn1
  Three-Phase V-I Measurementpt_1/RConn3 -- c/RConn1
  Three-Phase V-I Measurementpt_1/RConn2 -- b/RConn1

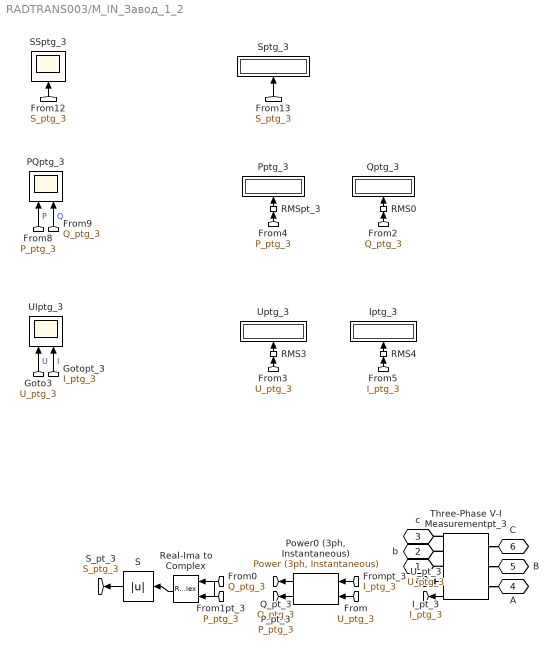
== system RADTRANS003/M_IN_Завод_1_2 ==
  Iptg_3 : Display
      settings: Format=bank
  PQptg_3 : Scope  NumInputPorts=2
  "Power0 (3ph, Instantaneous)" : powerlib_meascontrol/Measurements/Power (3ph, Instantaneous)
  Pptg_3 : Display
      settings: Format=bank
  Qptg_3 : Display
      settings: Format=bank
  RMS0 : dspstat3/RMS  run=off  directionMode=Each column  dimension=1  InputProcessing=Columns as channels (frame based)  reset_popup=None
  RMS3 : dspstat3/RMS  run=off  directionMode=Each column  dimension=1  InputProcessing=Columns as channels (frame based)  reset_popup=None
  RMS4 : dspstat3/RMS  run=off  directionMode=Each column  dimension=1  InputProcessing=Columns as channels (frame based)  reset_popup=None
  RMSpt_3 : dspstat3/RMS  run=off  directionMode=Each column  dimension=1  InputProcessing=Columns as channels (frame based)  reset_popup=None
  Real-Ima to Complex : RealImagToComplex
  S : Abs
  SSptg_3 : Scope
  Sptg_3 : Display
      settings: Format=bank
  Three-Phase V-I Measurementpt_3 : powerlib/Measurements/Three-Phase V-I Measurement  VoltageMeasurement=phase-to-ground  SetLabelV=off  LabelV=Vabc  Vpu=off  VpuLL=off  CurrentMeasurement=yes  SetLabelI=off  LabelI=Iabc  Ipu=off  Pbase=100e6  Vbase=500e3  OutputType=Complex  PhasorSimulation=off  PSBequivalent=0
  UIptg_3 : Scope  NumInputPorts=2
  Uptg_3 : Display
      settings: Format=bank
  a : PMIOPort  Side=Right
  b : PMIOPort  Port=2  Side=Right
  c : PMIOPort  Port=3  Side=Right
  A : PMIOPort  Port=4  Side=Left
  B : PMIOPort  Port=5  Side=Left
  C : PMIOPort  Port=6  Side=Left
  tag scope: I_ptg_3=global, P_ptg_3=global, Q_ptg_3=global, S_ptg_3=global, U_ptg_3=global
  wires:
  S/1 -> [S_ptg_3]
  Real-Ima to Complex/1 -> S/1
  [S_ptg_3] -> Sptg_3/1
  [S_ptg_3] -> SSptg_3/1
  [P_ptg_3] -> RMSpt_3/1
  RMSpt_3/1 -> Pptg_3/1
  RMS0/1 -> Qptg_3/1
  [U_ptg_3] -> RMS3/1
  RMS3/1 -> Uptg_3/1
  [P_ptg_3] -> Real-Ima to Complex/1
  [Q_ptg_3] -> RMS0/1
  [I_ptg_3] -> RMS4/1
  RMS4/1 -> Iptg_3/1
  [U_ptg_3] -> UIptg_3/1  "U"
  [P_ptg_3] -> PQptg_3/1  "P"
  [I_ptg_3] -> UIptg_3/2  "I"
  Three-Phase V-I Measurementpt_3/1 -> [U_ptg_3]
  [Q_ptg_3] -> Real-Ima to Complex/2
  Three-Phase V-I Measurementpt_3/2 -> [I_ptg_3]
  [U_ptg_3] -> "Power0 (3ph, Instantaneous)"/1
  [I_ptg_3] -> "Power0 (3ph, Instantaneous)"/2
  "Power0 (3ph, Instantaneous)"/2 -> [Q_ptg_3]
  "Power0 (3ph, Instantaneous)"/1 -> [P_ptg_3]
  [Q_ptg_3] -> PQptg_3/2  "Q"
  connections:
  Three-Phase V-I Measurementpt_3/LConn1 -- A/RConn1
  Three-Phase V-I Measurementpt_3/RConn1 -- a/RConn1
  Three-Phase V-I Measurementpt_3/LConn2 -- B/RConn1
  Three-Phase V-I Measurementpt_3/LConn3 -- C/RConn1
  Three-Phase V-I Measurementpt_3/RConn3 -- c/RConn1
  Three-Phase V-I Measurementpt_3/RConn2 -- b/RConn1

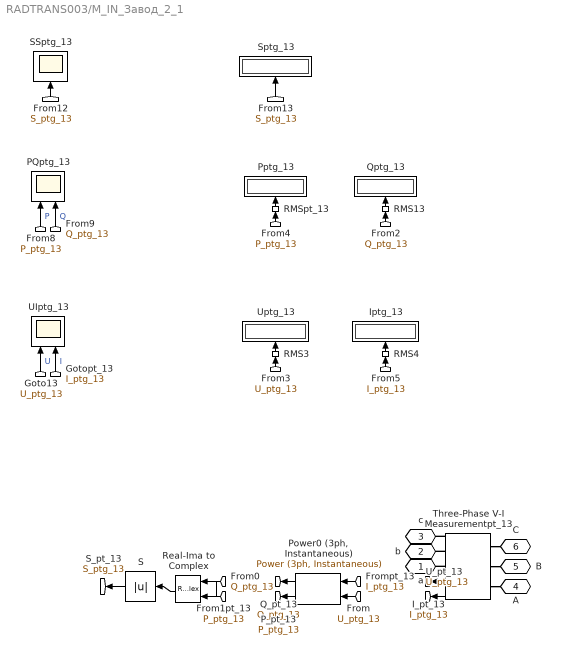
== system RADTRANS003/M_IN_Завод_2_1 ==
  Iptg_13 : Display
      settings: Format=bank
  PQptg_13 : Scope  NumInputPorts=2
  "Power0 (3ph, Instantaneous)" : powerlib_meascontrol/Measurements/Power (3ph, Instantaneous)
  Pptg_13 : Display
      settings: Format=bank
  Qptg_13 : Display
      settings: Format=bank
  RMS13 : dspstat3/RMS  run=off  directionMode=Each column  dimension=1  InputProcessing=Columns as channels (frame based)  reset_popup=None
  RMS3 : dspstat3/RMS  run=off  directionMode=Each column  dimension=1  InputProcessing=Columns as channels (frame based)  reset_popup=None
  RMS4 : dspstat3/RMS  run=off  directionMode=Each column  dimension=1  InputProcessing=Columns as channels (frame based)  reset_popup=None
  RMSpt_13 : dspstat3/RMS  run=off  directionMode=Each column  dimension=1  InputProcessing=Columns as channels (frame based)  reset_popup=None
  Real-Ima to Complex : RealImagToComplex
  S : Abs
  SSptg_13 : Scope
  Sptg_13 : Display
      settings: Format=bank
  Three-Phase V-I Measurementpt_13 : powerlib/Measurements/Three-Phase V-I Measurement  VoltageMeasurement=phase-to-ground  SetLabelV=off  LabelV=Vabc  Vpu=off  VpuLL=off  CurrentMeasurement=yes  SetLabelI=off  LabelI=Iabc  Ipu=off  Pbase=100e6  Vbase=500e3  OutputType=Complex  PhasorSimulation=off  PSBequivalent=0
  UIptg_13 : Scope  NumInputPorts=2
  Uptg_13 : Display
      settings: Format=bank
  a : PMIOPort  Side=Right
  b : PMIOPort  Port=2  Side=Right
  c : PMIOPort  Port=3  Side=Right
  A : PMIOPort  Port=4  Side=Left
  B : PMIOPort  Port=5  Side=Left
  C : PMIOPort  Port=6  Side=Left
  tag scope: I_ptg_13=global, P_ptg_13=global, Q_ptg_13=global, S_ptg_13=global, U_ptg_13=global
  wires:
  S/1 -> [S_ptg_13]
  Real-Ima to Complex/1 -> S/1
  [S_ptg_13] -> Sptg_13/1
  [S_ptg_13] -> SSptg_13/1
  [P_ptg_13] -> RMSpt_13/1
  RMSpt_13/1 -> Pptg_13/1
  RMS13/1 -> Qptg_13/1
  [U_ptg_13] -> RMS3/1
  RMS3/1 -> Uptg_13/1
  [P_ptg_13] -> Real-Ima to Complex/1
  [Q_ptg_13] -> RMS13/1
  [I_ptg_13] -> RMS4/1
  RMS4/1 -> Iptg_13/1
  [U_ptg_13] -> UIptg_13/1  "U"
  [P_ptg_13] -> PQptg_13/1  "P"
  [I_ptg_13] -> UIptg_13/2  "I"
  Three-Phase V-I Measurementpt_13/1 -> [U_ptg_13]
  [Q_ptg_13] -> Real-Ima to Complex/2
  Three-Phase V-I Measurementpt_13/2 -> [I_ptg_13]
  [U_ptg_13] -> "Power0 (3ph, Instantaneous)"/1
  [I_ptg_13] -> "Power0 (3ph, Instantaneous)"/2
  "Power0 (3ph, Instantaneous)"/2 -> [Q_ptg_13]
  "Power0 (3ph, Instantaneous)"/1 -> [P_ptg_13]
  [Q_ptg_13] -> PQptg_13/2  "Q"
  connections:
  Three-Phase V-I Measurementpt_13/LConn1 -- A/RConn1
  Three-Phase V-I Measurementpt_13/RConn1 -- a/RConn1
  Three-Phase V-I Measurementpt_13/LConn2 -- B/RConn1
  Three-Phase V-I Measurementpt_13/LConn3 -- C/RConn1
  Three-Phase V-I Measurementpt_13/RConn3 -- c/RConn1
  Three-Phase V-I Measurementpt_13/RConn2 -- b/RConn1

== system RADTRANS003/M_IN_Завод_2_2 ==
  Iptg_15 : Display
      settings: Format=bank
  PQptg_15 : Scope  NumInputPorts=2
  "Power0 (3ph, Instantaneous)" : powerlib_meascontrol/Measurements/Power (3ph, Instantaneous)
  Pptg_15 : Display
      settings: Format=bank
  Qptg_15 : Display
      settings: Format=bank
  RMS15 : dspstat3/RMS  run=off  directionMode=Each column  dimension=1  InputProcessing=Columns as channels (frame based)  reset_popup=None
  RMS3 : dspstat3/RMS  run=off  directionMode=Each column  dimension=1  InputProcessing=Columns as channels (frame based)  reset_popup=None
  RMS4 : dspstat3/RMS  run=off  directionMode=Each column  dimension=1  InputProcessing=Columns as channels (frame based)  reset_popup=None
  RMSpt_15 : dspstat3/RMS  run=off  directionMode=Each column  dimension=1  InputProcessing=Columns as channels (frame based)  reset_popup=None
  Real-Ima to Complex : RealImagToComplex
  S : Abs
  SSptg_15 : Scope
  Sptg_15 : Display
      settings: Format=bank
  Three-Phase V-I Measurementpt_15 : powerlib/Measurements/Three-Phase V-I Measurement  VoltageMeasurement=phase-to-ground  SetLabelV=off  LabelV=Vabc  Vpu=off  VpuLL=off  CurrentMeasurement=yes  SetLabelI=off  LabelI=Iabc  Ipu=off  Pbase=100e6  Vbase=500e3  OutputType=Complex  PhasorSimulation=off  PSBequivalent=0
  UIptg_15 : Scope  NumInputPorts=2
  Uptg_15 : Display
      settings: Format=bank
  a : PMIOPort  Side=Right
  b : PMIOPort  Port=2  Side=Right
  c : PMIOPort  Port=3  Side=Right
  A : PMIOPort  Port=4  Side=Left
  B : PMIOPort  Port=5  Side=Left
  C : PMIOPort  Port=6  Side=Left
  tag scope: I_ptg_15=global, P_ptg_15=global, Q_ptg_15=global, S_ptg_15=global, U_ptg_15=global
  wires:
  S/1 -> [S_ptg_15]
  Real-Ima to Complex/1 -> S/1
  [S_ptg_15] -> Sptg_15/1
  [S_ptg_15] -> SSptg_15/1
  [P_ptg_15] -> RMSpt_15/1
  RMSpt_15/1 -> Pptg_15/1
  RMS15/1 -> Qptg_15/1
  [U_ptg_15] -> RMS3/1
  RMS3/1 -> Uptg_15/1
  [P_ptg_15] -> Real-Ima to Complex/1
  [Q_ptg_15] -> RMS15/1
  [I_ptg_15] -> RMS4/1
  RMS4/1 -> Iptg_15/1
  [U_ptg_15] -> UIptg_15/1  "U"
  [P_ptg_15] -> PQptg_15/1  "P"
  [I_ptg_15] -> UIptg_15/2  "I"
  Three-Phase V-I Measurementpt_15/1 -> [U_ptg_15]
  [Q_ptg_15] -> Real-Ima to Complex/2
  Three-Phase V-I Measurementpt_15/2 -> [I_ptg_15]
  [U_ptg_15] -> "Power0 (3ph, Instantaneous)"/1
  [I_ptg_15] -> "Power0 (3ph, Instantaneous)"/2
  "Power0 (3ph, Instantaneous)"/2 -> [Q_ptg_15]
  "Power0 (3ph, Instantaneous)"/1 -> [P_ptg_15]
  [Q_ptg_15] -> PQptg_15/2  "Q"
  connections:
  Three-Phase V-I Measurementpt_15/LConn1 -- A/RConn1
  Three-Phase V-I Measurementpt_15/RConn1 -- a/RConn1
  Three-Phase V-I Measurementpt_15/LConn2 -- B/RConn1
  Three-Phase V-I Measurementpt_15/LConn3 -- C/RConn1
  Three-Phase V-I Measurementpt_15/RConn3 -- c/RConn1
  Three-Phase V-I Measurementpt_15/RConn2 -- b/RConn1

== system RADTRANS003/M_OUT_Город_1_1 ==
  Iptg_6 : Display
      settings: Format=bank
  PQptg_6 : Scope  NumInputPorts=2
  "Power0 (3ph, Instantaneous)" : powerlib_meascontrol/Measurements/Power (3ph, Instantaneous)
  Pptg_6 : Display
      settings: Format=bank
  Qptg_6 : Display
      settings: Format=bank
  RMS3 : dspstat3/RMS  run=off  directionMode=Each column  dimension=1  InputProcessing=Columns as channels (frame based)  reset_popup=None
  RMS4 : dspstat3/RMS  run=off  directionMode=Each column  dimension=1  InputProcessing=Columns as channels (frame based)  reset_popup=None
  RMS6 : dspstat3/RMS  run=off  directionMode=Each column  dimension=1  InputProcessing=Columns as channels (frame based)  reset_popup=None
  RMSpt_6 : dspstat3/RMS  run=off  directionMode=Each column  dimension=1  InputProcessing=Columns as channels (frame based)  reset_popup=None
  Real-Ima to Complex : RealImagToComplex
  S : Abs
  SSptg_6 : Scope
  Sptg_6 : Display
      settings: Format=bank
  Three-Phase V-I Measurementpt_6 : powerlib/Measurements/Three-Phase V-I Measurement  VoltageMeasurement=phase-to-ground  SetLabelV=off  LabelV=Vabc  Vpu=off  VpuLL=off  CurrentMeasurement=yes  SetLabelI=off  LabelI=Iabc  Ipu=off  Pbase=100e6  Vbase=500e3  OutputType=Complex  PhasorSimulation=off  PSBequivalent=0
  UIptg_6 : Scope  NumInputPorts=2
  Uptg_6 : Display
      settings: Format=bank
  a : PMIOPort  Side=Right
  b : PMIOPort  Port=2  Side=Right
  c : PMIOPort  Port=3  Side=Right
  A : PMIOPort  Port=4  Side=Left
  B : PMIOPort  Port=5  Side=Left
  C : PMIOPort  Port=6  Side=Left
  tag scope: I_ptg_6=global, P_ptg_6=global, Q_ptg_6=global, S_ptg_6=global, U_ptg_6=global
  wires:
  S/1 -> [S_ptg_6]
  Real-Ima to Complex/1 -> S/1
  [S_ptg_6] -> Sptg_6/1
  [S_ptg_6] -> SSptg_6/1
  [P_ptg_6] -> RMSpt_6/1
  RMSpt_6/1 -> Pptg_6/1
  RMS6/1 -> Qptg_6/1
  [U_ptg_6] -> RMS3/1
  RMS3/1 -> Uptg_6/1
  [P_ptg_6] -> Real-Ima to Complex/1
  [Q_ptg_6] -> RMS6/1
  [I_ptg_6] -> RMS4/1
  RMS4/1 -> Iptg_6/1
  [U_ptg_6] -> UIptg_6/1  "U"
  [P_ptg_6] -> PQptg_6/1  "P"
  [I_ptg_6] -> UIptg_6/2  "I"
  Three-Phase V-I Measurementpt_6/1 -> [U_ptg_6]
  [Q_ptg_6] -> Real-Ima to Complex/2
  Three-Phase V-I Measurementpt_6/2 -> [I_ptg_6]
  [U_ptg_6] -> "Power0 (3ph, Instantaneous)"/1
  [I_ptg_6] -> "Power0 (3ph, Instantaneous)"/2
  "Power0 (3ph, Instantaneous)"/2 -> [Q_ptg_6]
  "Power0 (3ph, Instantaneous)"/1 -> [P_ptg_6]
  [Q_ptg_6] -> PQptg_6/2  "Q"
  connections:
  Three-Phase V-I Measurementpt_6/LConn1 -- A/RConn1
  Three-Phase V-I Measurementpt_6/RConn1 -- a/RConn1
  Three-Phase V-I Measurementpt_6/LConn2 -- B/RConn1
  Three-Phase V-I Measurementpt_6/LConn3 -- C/RConn1
  Three-Phase V-I Measurementpt_6/RConn3 -- c/RConn1
  Three-Phase V-I Measurementpt_6/RConn2 -- b/RConn1

== system RADTRANS003/M_OUT_Город_1_2 ==
  Iptg_8 : Display
      settings: Format=bank
  PQptg_8 : Scope  NumInputPorts=2
  "Power0 (3ph, Instantaneous)" : powerlib_meascontrol/Measurements/Power (3ph, Instantaneous)
  Pptg_8 : Display
      settings: Format=bank
  Qptg_8 : Display
      settings: Format=bank
  RMS3 : dspstat3/RMS  run=off  directionMode=Each column  dimension=1  InputProcessing=Columns as channels (frame based)  reset_popup=None
  RMS4 : dspstat3/RMS  run=off  directionMode=Each column  dimension=1  InputProcessing=Columns as channels (frame based)  reset_popup=None
  RMS8 : dspstat3/RMS  run=off  directionMode=Each column  dimension=1  InputProcessing=Columns as channels (frame based)  reset_popup=None
  RMSpt_8 : dspstat3/RMS  run=off  directionMode=Each column  dimension=1  InputProcessing=Columns as channels (frame based)  reset_popup=None
  Real-Ima to Complex : RealImagToComplex
  S : Abs
  SSptg_8 : Scope
  Sptg_8 : Display
      settings: Format=bank
  Three-Phase V-I Measurementpt_8 : powerlib/Measurements/Three-Phase V-I Measurement  VoltageMeasurement=phase-to-ground  SetLabelV=off  LabelV=Vabc  Vpu=off  VpuLL=off  CurrentMeasurement=yes  SetLabelI=off  LabelI=Iabc  Ipu=off  Pbase=100e6  Vbase=500e3  OutputType=Complex  PhasorSimulation=off  PSBequivalent=0
  UIptg_8 : Scope  NumInputPorts=2
  Uptg_8 : Display
      settings: Format=bank
  a : PMIOPort  Side=Right
  b : PMIOPort  Port=2  Side=Right
  c : PMIOPort  Port=3  Side=Right
  A : PMIOPort  Port=4  Side=Left
  B : PMIOPort  Port=5  Side=Left
  C : PMIOPort  Port=6  Side=Left
  tag scope: I_ptg_8=global, P_ptg_8=global, Q_ptg_8=global, S_ptg_8=global, U_ptg_8=global
  wires:
  S/1 -> [S_ptg_8]
  Real-Ima to Complex/1 -> S/1
  [S_ptg_8] -> Sptg_8/1
  [S_ptg_8] -> SSptg_8/1
  [P_ptg_8] -> RMSpt_8/1
  RMSpt_8/1 -> Pptg_8/1
  RMS8/1 -> Qptg_8/1
  [U_ptg_8] -> RMS3/1
  RMS3/1 -> Uptg_8/1
  [P_ptg_8] -> Real-Ima to Complex/1
  [Q_ptg_8] -> RMS8/1
  [I_ptg_8] -> RMS4/1
  RMS4/1 -> Iptg_8/1
  [U_ptg_8] -> UIptg_8/1  "U"
  [P_ptg_8] -> PQptg_8/1  "P"
  [I_ptg_8] -> UIptg_8/2  "I"
  Three-Phase V-I Measurementpt_8/1 -> [U_ptg_8]
  [Q_ptg_8] -> Real-Ima to Complex/2
  Three-Phase V-I Measurementpt_8/2 -> [I_ptg_8]
  [U_ptg_8] -> "Power0 (3ph, Instantaneous)"/1
  [I_ptg_8] -> "Power0 (3ph, Instantaneous)"/2
  "Power0 (3ph, Instantaneous)"/2 -> [Q_ptg_8]
  "Power0 (3ph, Instantaneous)"/1 -> [P_ptg_8]
  [Q_ptg_8] -> PQptg_8/2  "Q"
  connections:
  Three-Phase V-I Measurementpt_8/LConn1 -- A/RConn1
  Three-Phase V-I Measurementpt_8/RConn1 -- a/RConn1
  Three-Phase V-I Measurementpt_8/LConn2 -- B/RConn1
  Three-Phase V-I Measurementpt_8/LConn3 -- C/RConn1
  Three-Phase V-I Measurementpt_8/RConn3 -- c/RConn1
  Three-Phase V-I Measurementpt_8/RConn2 -- b/RConn1

== system RADTRANS003/M_OUT_Город_1_3 ==
  Iptg_10 : Display
      settings: Format=bank
  PQptg_10 : Scope  NumInputPorts=2
  "Power0 (3ph, Instantaneous)" : powerlib_meascontrol/Measurements/Power (3ph, Instantaneous)
  Pptg_10 : Display
      settings: Format=bank
  Qptg_10 : Display
      settings: Format=bank
  RMS10 : dspstat3/RMS  run=off  directionMode=Each column  dimension=1  InputProcessing=Columns as channels (frame based)  reset_popup=None
  RMS3 : dspstat3/RMS  run=off  directionMode=Each column  dimension=1  InputProcessing=Columns as channels (frame based)  reset_popup=None
  RMS4 : dspstat3/RMS  run=off  directionMode=Each column  dimension=1  InputProcessing=Columns as channels (frame based)  reset_popup=None
  RMSpt_10 : dspstat3/RMS  run=off  directionMode=Each column  dimension=1  InputProcessing=Columns as channels (frame based)  reset_popup=None
  Real-Ima to Complex : RealImagToComplex
  S : Abs
  SSptg_10 : Scope
  Sptg_10 : Display
      settings: Format=bank
  Three-Phase V-I Measurementpt_10 : powerlib/Measurements/Three-Phase V-I Measurement  VoltageMeasurement=phase-to-ground  SetLabelV=off  LabelV=Vabc  Vpu=off  VpuLL=off  CurrentMeasurement=yes  SetLabelI=off  LabelI=Iabc  Ipu=off  Pbase=100e6  Vbase=500e3  OutputType=Complex  PhasorSimulation=off  PSBequivalent=0
  UIptg_10 : Scope  NumInputPorts=2
  Uptg_10 : Display
      settings: Format=bank
  a : PMIOPort  Side=Right
  b : PMIOPort  Port=2  Side=Right
  c : PMIOPort  Port=3  Side=Right
  A : PMIOPort  Port=4  Side=Left
  B : PMIOPort  Port=5  Side=Left
  C : PMIOPort  Port=6  Side=Left
  tag scope: I_ptg_10=global, P_ptg_10=global, Q_ptg_10=global, S_ptg_10=global, U_ptg_10=global
  wires:
  S/1 -> [S_ptg_10]
  Real-Ima to Complex/1 -> S/1
  [S_ptg_10] -> Sptg_10/1
  [S_ptg_10] -> SSptg_10/1
  [P_ptg_10] -> RMSpt_10/1
  RMSpt_10/1 -> Pptg_10/1
  RMS10/1 -> Qptg_10/1
  [U_ptg_10] -> RMS3/1
  RMS3/1 -> Uptg_10/1
  [P_ptg_10] -> Real-Ima to Complex/1
  [Q_ptg_10] -> RMS10/1
  [I_ptg_10] -> RMS4/1
  RMS4/1 -> Iptg_10/1
  [U_ptg_10] -> UIptg_10/1  "U"
  [P_ptg_10] -> PQptg_10/1  "P"
  [I_ptg_10] -> UIptg_10/2  "I"
  Three-Phase V-I Measurementpt_10/1 -> [U_ptg_10]
  [Q_ptg_10] -> Real-Ima to Complex/2
  Three-Phase V-I Measurementpt_10/2 -> [I_ptg_10]
  [U_ptg_10] -> "Power0 (3ph, Instantaneous)"/1
  [I_ptg_10] -> "Power0 (3ph, Instantaneous)"/2
  "Power0 (3ph, Instantaneous)"/2 -> [Q_ptg_10]
  "Power0 (3ph, Instantaneous)"/1 -> [P_ptg_10]
  [Q_ptg_10] -> PQptg_10/2  "Q"
  connections:
  Three-Phase V-I Measurementpt_10/LConn1 -- A/RConn1
  Three-Phase V-I Measurementpt_10/RConn1 -- a/RConn1
  Three-Phase V-I Measurementpt_10/LConn2 -- B/RConn1
  Three-Phase V-I Measurementpt_10/LConn3 -- C/RConn1
  Three-Phase V-I Measurementpt_10/RConn3 -- c/RConn1
  Three-Phase V-I Measurementpt_10/RConn2 -- b/RConn1

== system RADTRANS003/M_OUT_Город_1_4 ==
  Iptg_12 : Display
      settings: Format=bank
  PQptg_12 : Scope  NumInputPorts=2
  "Power0 (3ph, Instantaneous)" : powerlib_meascontrol/Measurements/Power (3ph, Instantaneous)
  Pptg_12 : Display
      settings: Format=bank
  Qptg_12 : Display
      settings: Format=bank
  RMS12 : dspstat3/RMS  run=off  directionMode=Each column  dimension=1  InputProcessing=Columns as channels (frame based)  reset_popup=None
  RMS3 : dspstat3/RMS  run=off  directionMode=Each column  dimension=1  InputProcessing=Columns as channels (frame based)  reset_popup=None
  RMS4 : dspstat3/RMS  run=off  directionMode=Each column  dimension=1  InputProcessing=Columns as channels (frame based)  reset_popup=None
  RMSpt_12 : dspstat3/RMS  run=off  directionMode=Each column  dimension=1  InputProcessing=Columns as channels (frame based)  reset_popup=None
  Real-Ima to Complex : RealImagToComplex
  S : Abs
  SSptg_12 : Scope
  Sptg_12 : Display
      settings: Format=bank
  Three-Phase V-I Measurementpt_12 : powerlib/Measurements/Three-Phase V-I Measurement  VoltageMeasurement=phase-to-ground  SetLabelV=off  LabelV=Vabc  Vpu=off  VpuLL=off  CurrentMeasurement=yes  SetLabelI=off  LabelI=Iabc  Ipu=off  Pbase=100e6  Vbase=500e3  OutputType=Complex  PhasorSimulation=off  PSBequivalent=0
  UIptg_12 : Scope  NumInputPorts=2
  Uptg_12 : Display
      settings: Format=bank
  a : PMIOPort  Side=Right
  b : PMIOPort  Port=2  Side=Right
  c : PMIOPort  Port=3  Side=Right
  A : PMIOPort  Port=4  Side=Left
  B : PMIOPort  Port=5  Side=Left
  C : PMIOPort  Port=6  Side=Left
  tag scope: I_ptg_12=global, P_ptg_12=global, Q_ptg_12=global, S_ptg_12=global, U_ptg_12=global
  wires:
  S/1 -> [S_ptg_12]
  Real-Ima to Complex/1 -> S/1
  [S_ptg_12] -> Sptg_12/1
  [S_ptg_12] -> SSptg_12/1
  [P_ptg_12] -> RMSpt_12/1
  RMSpt_12/1 -> Pptg_12/1
  RMS12/1 -> Qptg_12/1
  [U_ptg_12] -> RMS3/1
  RMS3/1 -> Uptg_12/1
  [P_ptg_12] -> Real-Ima to Complex/1
  [Q_ptg_12] -> RMS12/1
  [I_ptg_12] -> RMS4/1
  RMS4/1 -> Iptg_12/1
  [U_ptg_12] -> UIptg_12/1  "U"
  [P_ptg_12] -> PQptg_12/1  "P"
  [I_ptg_12] -> UIptg_12/2  "I"
  Three-Phase V-I Measurementpt_12/1 -> [U_ptg_12]
  [Q_ptg_12] -> Real-Ima to Complex/2
  Three-Phase V-I Measurementpt_12/2 -> [I_ptg_12]
  [U_ptg_12] -> "Power0 (3ph, Instantaneous)"/1
  [I_ptg_12] -> "Power0 (3ph, Instantaneous)"/2
  "Power0 (3ph, Instantaneous)"/2 -> [Q_ptg_12]
  "Power0 (3ph, Instantaneous)"/1 -> [P_ptg_12]
  [Q_ptg_12] -> PQptg_12/2  "Q"
  connections:
  Three-Phase V-I Measurementpt_12/LConn1 -- A/RConn1
  Three-Phase V-I Measurementpt_12/RConn1 -- a/RConn1
  Three-Phase V-I Measurementpt_12/LConn2 -- B/RConn1
  Three-Phase V-I Measurementpt_12/LConn3 -- C/RConn1
  Three-Phase V-I Measurementpt_12/RConn3 -- c/RConn1
  Three-Phase V-I Measurementpt_12/RConn2 -- b/RConn1

== system RADTRANS003/M_OUT_Город_2_1 ==
  Iptg_18 : Display
      settings: Format=bank
  PQptg_18 : Scope  NumInputPorts=2
  "Power0 (3ph, Instantaneous)" : powerlib_meascontrol/Measurements/Power (3ph, Instantaneous)
  Pptg_18 : Display
      settings: Format=bank
  Qptg_18 : Display
      settings: Format=bank
  RMS18 : dspstat3/RMS  run=off  directionMode=Each column  dimension=1  InputProcessing=Columns as channels (frame based)  reset_popup=None
  RMS3 : dspstat3/RMS  run=off  directionMode=Each column  dimension=1  InputProcessing=Columns as channels (frame based)  reset_popup=None
  RMS4 : dspstat3/RMS  run=off  directionMode=Each column  dimension=1  InputProcessing=Columns as channels (frame based)  reset_popup=None
  RMSpt_18 : dspstat3/RMS  run=off  directionMode=Each column  dimension=1  InputProcessing=Columns as channels (frame based)  reset_popup=None
  Real-Ima to Complex : RealImagToComplex
  S : Abs
  SSptg_18 : Scope
  Sptg_18 : Display
      settings: Format=bank
  Three-Phase V-I Measurementpt_18 : powerlib/Measurements/Three-Phase V-I Measurement  VoltageMeasurement=phase-to-ground  SetLabelV=off  LabelV=Vabc  Vpu=off  VpuLL=off  CurrentMeasurement=yes  SetLabelI=off  LabelI=Iabc  Ipu=off  Pbase=100e6  Vbase=500e3  OutputType=Complex  PhasorSimulation=off  PSBequivalent=0
  UIptg_18 : Scope  NumInputPorts=2
  Uptg_18 : Display
      settings: Format=bank
  a : PMIOPort  Side=Right
  b : PMIOPort  Port=2  Side=Right
  c : PMIOPort  Port=3  Side=Right
  A : PMIOPort  Port=4  Side=Left
  B : PMIOPort  Port=5  Side=Left
  C : PMIOPort  Port=6  Side=Left
  tag scope: I_ptg_18=global, P_ptg_18=global, Q_ptg_18=global, S_ptg_18=global, U_ptg_18=global
  wires:
  S/1 -> [S_ptg_18]
  Real-Ima to Complex/1 -> S/1
  [S_ptg_18] -> Sptg_18/1
  [S_ptg_18] -> SSptg_18/1
  [P_ptg_18] -> RMSpt_18/1
  RMSpt_18/1 -> Pptg_18/1
  RMS18/1 -> Qptg_18/1
  [U_ptg_18] -> RMS3/1
  RMS3/1 -> Uptg_18/1
  [P_ptg_18] -> Real-Ima to Complex/1
  [Q_ptg_18] -> RMS18/1
  [I_ptg_18] -> RMS4/1
  RMS4/1 -> Iptg_18/1
  [U_ptg_18] -> UIptg_18/1  "U"
  [P_ptg_18] -> PQptg_18/1  "P"
  [I_ptg_18] -> UIptg_18/2  "I"
  Three-Phase V-I Measurementpt_18/1 -> [U_ptg_18]
  [Q_ptg_18] -> Real-Ima to Complex/2
  Three-Phase V-I Measurementpt_18/2 -> [I_ptg_18]
  [U_ptg_18] -> "Power0 (3ph, Instantaneous)"/1
  [I_ptg_18] -> "Power0 (3ph, Instantaneous)"/2
  "Power0 (3ph, Instantaneous)"/2 -> [Q_ptg_18]
  "Power0 (3ph, Instantaneous)"/1 -> [P_ptg_18]
  [Q_ptg_18] -> PQptg_18/2  "Q"
  connections:
  Three-Phase V-I Measurementpt_18/LConn1 -- A/RConn1
  Three-Phase V-I Measurementpt_18/RConn1 -- a/RConn1
  Three-Phase V-I Measurementpt_18/LConn2 -- B/RConn1
  Three-Phase V-I Measurementpt_18/LConn3 -- C/RConn1
  Three-Phase V-I Measurementpt_18/RConn3 -- c/RConn1
  Three-Phase V-I Measurementpt_18/RConn2 -- b/RConn1
